simulink model "EKF_Known"  (R2020b)
settings: Solver=ode45  StartTime=0.0  StopTime=200  FixedStep=1e-7  RelTol=1e-4  AbsTol=1e-4  EnableMultiTasking=on
settings Model: Creator=André  LastModifiedBy=Andre
settings SolverCC: AutoScaleAbsTol=off  ConsecutiveZCsStepRelTol=100*128*eps  ShapePreserveControl=EnableAll  ZeroCrossControl=EnableAll  AutoInsertRateTranBlk=on
settings DataIOCC: LimitDataPoints=on  SaveFormat=Array  SignalLoggingSaveFormat=ModelDataLogs  ReturnWorkspaceOutputs=off
settings OptimizationCC: ExpressionDepthLimit=2147483647  LifeSpan=inf
settings DebuggingCC: UnderspecifiedInitializationDetection=Classic  MergeDetectMultiDrivingBlocksExec=none  SolverPrmCheckMsg=warning  FcnCallInpInsideContextMsg=warning  StateNameClashWarn=warning  SFUnexpectedBacktrackingDiag=warning  SFNoUnconditionalDefaultTransitionDiag=warning  SFExecutionAtInitializationDiag=none  ArithmeticOperatorsInVariantConditions=warning
settings HardwareCC: ProdBitPerPointer=32  ProdBitPerSizeT=32  ProdBitPerPtrDiffT=32  ProdLargestAtomicFloat=None  ProdIntDivRoundTo=Undefined  ProdEndianess=Unspecified  ProdWordSize=32  ProdHWDeviceType=32-bit Generic
settings ModelReferenceCC: PropagateSignalLabelsOutOfModel=off
settings SFSimCC: SimUseLocalCustomCode=off  SimParseCustomCode=off  CustomCodeUndefinedFunction=UseInterfaceOnly
settings RTWCC: RTWUseLocalCustomCode=off
settings CodeAppCC: StateflowObjectComments=on
settings GRTTargetCC: TargetLangStandard=C89/C90 (ANSI)  CombineOutputUpdateFcns=off  GRTInterface=on
settings ConfigComp: CovMetricSettings=dw  CovSaveCumulativeToWorkspaceVar=on  CovSaveSingleToWorkspaceVar=on  CovExternalEMLEnable=off

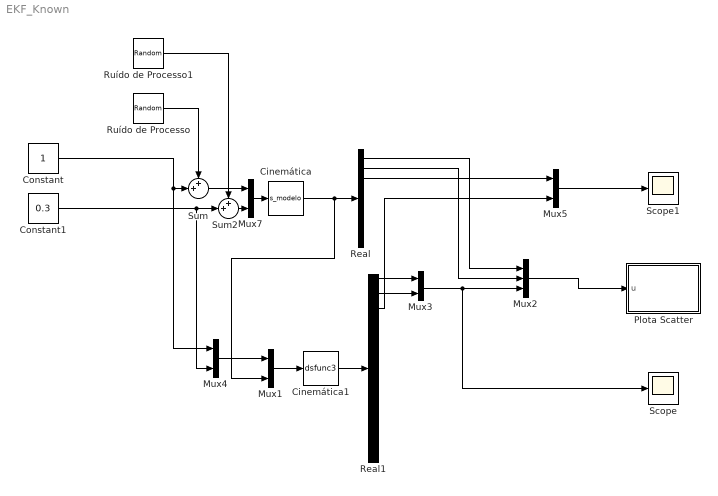
== system EKF_Known ==
  Cinemática : S-Function  FunctionName=s_modelo  Parameters=[0 -10 0]  SFunctionDeploymentMode=off  EnableBusSupport=off
  Cinemática1 : S-Function  FunctionName=dsfunc3  Parameters=[1 2 0 10 0 0 0 10 0 0 0 10 0]  SFunctionDeploymentMode=off  EnableBusSupport=off
  Constant : Constant
  Constant1 : Constant  Value=0.3
  Mux{1,3..5,7} (5 alike) : Mux  Inputs=2
  Mux2 : Mux  Inputs=3
  Plota Scatter : MATLAB Function  TreatAsAtomicUnit=on
  Real : Demux  Outputs=9
  Real1 : Demux  Outputs=13
  Ruído de Processo : RandomNumber  Variance=0.1  SampleTime=0.1
  Ruído de Processo1 : RandomNumber  Variance=0.1  SampleTime=0.1
  Scope : Scope
  Scope1 : Scope
  Sum : Sum  Inputs=++|
  Sum2 : Sum  Inputs=++|
  wires:
  Mux1/1 -> Cinemática1/1
  Ruído de Processo/1 -> Sum/1
  Mux7/1 -> Cinemática/1
  Sum2/1 -> Mux7/2
  Constant/1 -> Mux4/1, Sum/2
  Sum/1 -> Mux7/1
  Mux4/1 -> Mux1/1
  Cinemática/1 -> Mux1/2, Real/1
  Constant1/1 -> Mux4/2, Sum2/2
  Ruído de Processo1/1 -> Sum2/1
  Real/1 -> Mux2/1
  Real/2 -> Mux2/2
  Mux2/1 -> Plota Scatter/1(u)
  Cinemática1/1 -> Real1/1
  Mux3/1 -> Scope/1, Mux2/3
  Real1/3 -> Mux5/2
  Real1/1 -> Mux3/1
  Real1/2 -> Mux3/2
  Real/3 -> Mux5/1
  Mux5/1 -> Scope1/1

== matlab function EKF_Known/Plota Scatter ==
  data: u input
function  fcn(u)
     %n_Particulas = 1000;  
     %global marker
     marker = [-10 10; 10 10]; % Positions of markers  % Positions of markers
     %n_estados = n_Particulas*3;
     x = u(1:2);
     xx = u(3:4);
     %particulas = u(3:(2+n_estados));
     coder.extrinsic('scatter')
     
     
      %xP = reshape(particulas,3,[]);
      %x_ = mean(xP, 2);
      %x_ = u(3+n_estados:5+n_estados);
      %scatter(xP(1,:),xP(2,:), 'k.');
      axis( [-10 10 -10 10]);
      hold on;
      scatter(xx(1),xx(2),'bo');
      scatter(marker(:,1),marker(:,2), 'gs');
      scatter(x(1),x(2), 'r*');
      hold off;
     % insert additional code as needed to turn on grid, setup axis limits, etc.

  %%%%%%%%%
%y = u;
